simulink model "s_func"  (R2014a)
settings: Solver=ode3  SolverMode=MultiTasking  StartTime=0.0  StopTime=10  FixedStep=0.005  RelTol=1e-3
settings Model: Creator=atlabor  LastModifiedBy=Steffen

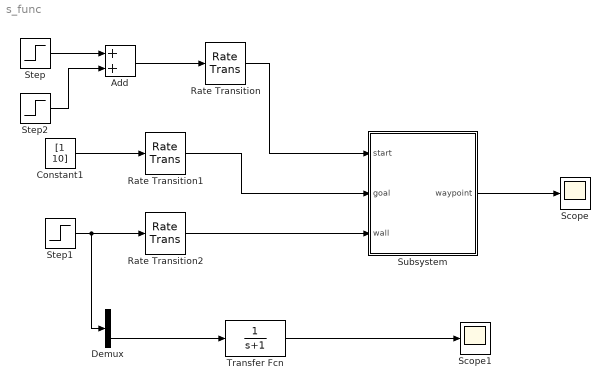
== system s_func ==
  Add : Sum
  Constant1 : Constant  Value=[1 10]
  Demux : Demux  Outputs=3
  Rate Transition : RateTransition  OutPortSampleTime=1
  Rate Transition1 : RateTransition  OutPortSampleTime=1
  Rate Transition2 : RateTransition  OutPortSampleTime=1
  Scope : Scope
  Scope1 : Scope
  Step : Step  Time=2  Before=[1 1]  After=[2 2]  SampleTime=0
  Step1 : Step  Time=3  Before=[0 0 0]  After=[1 3 1]  SampleTime=0
  Step2 : Step  Time=3  Before=[0 0]  After=[1 1]  SampleTime=0
  Subsystem : Subsystem
  Transfer Fcn : TransferFcn  Denominator=[1 1]
  wires:
  Constant1/1 -> Rate Transition1/1
  Step1/1 -> Demux/1, Rate Transition2/1
  Subsystem/1(waypoint) -> Scope/1
  Rate Transition/1 -> Subsystem/1(start)
  Rate Transition1/1 -> Subsystem/2(goal)
  Rate Transition2/1 -> Subsystem/3(wall)
  Transfer Fcn/1 -> Scope1/1
  Demux/3 -> Transfer Fcn/1
  Step/1 -> Add/1
  Step2/1 -> Add/2
  Add/1 -> Rate Transition/1

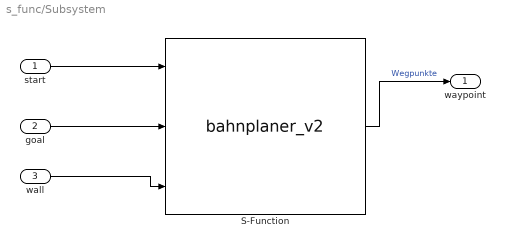
== system s_func/Subsystem ==
  start : Inport
  goal : Inport  Port=2
  wall : Inport  Port=3
  S-Function : S-Function  FunctionName=bahnplaner_v2  EnableBusSupport=off
      mask Display:
      | color('green');
      | port_label('input',1,'start (u1)');
      | port_label('input',2,'goal (u2)');
      | port_label('input',3,'wall (u3)');
      | color('black');
      | disp('Bahnplaner');
      | color('green');
      | port_label('output',1,'waypoints (y)');
  waypoint : Outport
  wires:
  goal/1 -> S-Function/2
  start/1 -> S-Function/1
  S-Function/1 -> waypoint/1  "Wegpunkte"
  wall/1 -> S-Function/3
